simulink model "single_phase_half_wave_controlled_rectifier"  (R2024a)
settings: Solver=VariableStepAuto  StartTime=0.0  StopTime=0.1  RelTol=1e-3
libraries: spsRMSLib x3, spsCurrentMeasurementLib x2, spsVoltageMeasurementLib x2, spsMeanLib x1, spsSeriesRLCBranchLib x1, spsThyristorLib x1, spsACVoltageSourceLib x1, spspowerguiLib x1
settings Model: Creator=Asus  LastModifiedBy=Asus

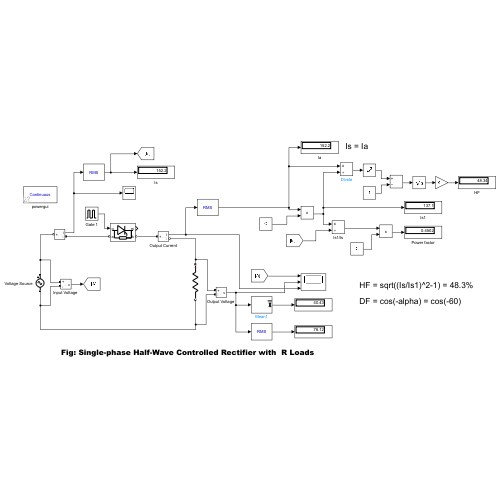
[thumbnail: Simulink's stored preview of the top-level diagram]
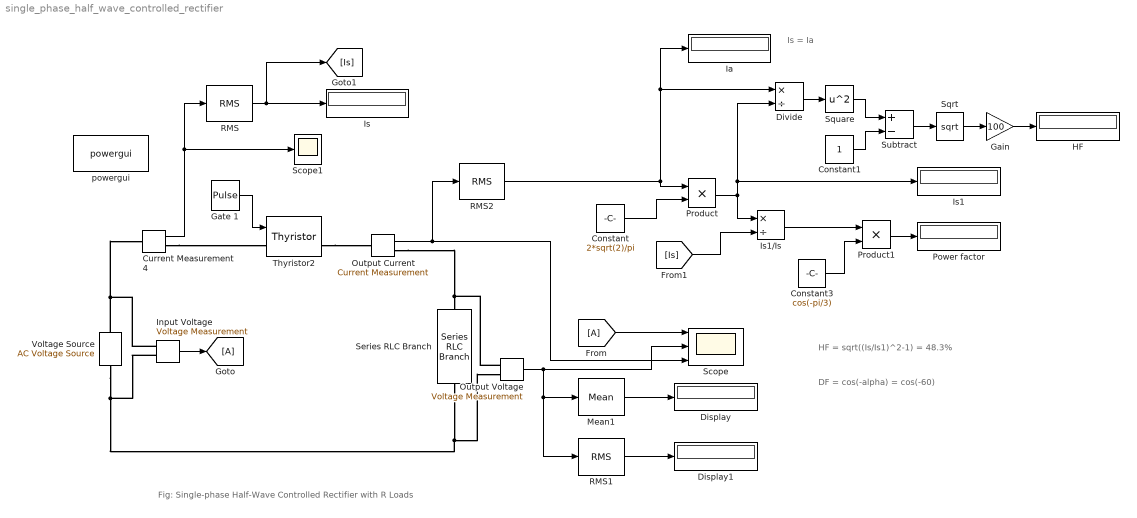
== system single_phase_half_wave_controlled_rectifier ==
  note: Is = Ia
  note: Fig: Single-phase Half-Wave Controlled Rectifier with R Loads
  note: HF = sqrt((Is/Is1)^2-1) = 48.3%
  note: DF = cos(-alpha) = cos(-60)
  Constant : Constant  Value=2*sqrt(2)/pi
  Constant1 : Constant
  Constant3 : Constant  Value=cos(-pi/3)
  Current Measurement4 : spsCurrentMeasurementLib/Current Measurement  PhasorSimulation=off  OutputType=Complex  PSBequivalent=0
  Display : Display
  Display1 : Display
  Divide : Product  Inputs=*/
  From : From
  Gain : Gain  Gain=100
  Gate 1 : DiscretePulseGenerator  PulseType=Time based  Period=1/60  PulseWidth=5  PhaseDelay=0.00277
  Goto : Goto
  HF : Display
  Ia : Display
  "Input Voltage " : spsVoltageMeasurementLib/Voltage Measurement  PhasorSimulation=off  OutputType=Complex  PSBequivalent=0
  Is : Display
  "Is1 " : Display
  Is1/Is : Product  Inputs=*/
  Mean1 : spsMeanLib/Mean  Freq=60  Vinit=0  Ts=0
  Output Current : spsCurrentMeasurementLib/Current Measurement  PhasorSimulation=off  OutputType=Complex  PSBequivalent=0
  "Output Voltage " : spsVoltageMeasurementLib/Voltage Measurement  PhasorSimulation=off  OutputType=Complex  PSBequivalent=0
  Power factor : Display
  Product : Product
  Product1 : Product
  RMS : spsRMSLib/RMS  TrueRMS=on  Freq=60  RMSInit=120  Ts=0
  RMS1 : spsRMSLib/RMS  TrueRMS=on  Freq=60  RMSInit=120  Ts=0
  RMS2 : spsRMSLib/RMS  TrueRMS=on  Freq=60  RMSInit=120  Ts=0
  Scope : Scope  NumInputPorts=3
  Scope1 : Scope
  Series RLC Branch : spsSeriesRLCBranchLib/Series RLC Branch  LConnTagsString=__new0  RConnTagsString=__new0  BranchType=R  Resistance=0.5  Inductance=6.5e-3  SetiL0=off  InitialCurrent=0  Capacitance=1e-6  Setx0=off  InitialVoltage=0  Measurements=None
  Sqrt : Sqrt
  Square : Math  Operator=square  SignedPower=on
  Subtract : Sum  Inputs=+-
  Thyristor2 : spsThyristorLib/Thyristor  Ron=0  Lon=0  Vf=0.1  IC=0  Rs=500  Cs=250e-9  Measurements=on
  Voltage Source : spsACVoltageSourceLib/AC Voltage Source  Amplitude=120*sqrt(2)  Phase=0  Frequency=60  SampleTime=0  Measurements=None  BusType=swing  Pref=10e3  Qref=0  Qmin=-inf  Qmax=+inf
  powergui : spspowerguiLib/powergui  Priority=1  SimulationMode=Continuous  SampleTime=50e-6  frequency=60  Iterations=50  frequencyindice=0  Pbase=100e6  ErrMax=1e-4  UnitsV=kV  UnitsW=MW  buscounter=0  FunctionMessages=off  echomessages=off  EnableUseOfTLC=off  CurrentSourceSwitches=off  DisableSnubberDevices=off  DisableRonSwitches=off  DisableVfSwitches=off  DisplayEquations=off  AutomaticDiscreteSolvers=off  SolverType=Tustin/Backward Euler (TBE)  Interpol=off  ExternalGateDelay=off  methode=off  Ts=100  x0status=blocks  SPID=on  SwTol=0  HookPort=off  NonlinearTolerance=0  nMaxIteration=15  ContinueOnMaxIteration=off  RestoreLinks=warning  ResistiveCurrentMeasurement=off  Frange=[0:2:500]  Ylog=off  Xlog=on  ShowGrid=off  save=off  variable=ZData  structure=p  ZoomFFT=off  StartTime=0.0  cycles=1  DisplayStyle=1  fundamental=60  FreqAxis=off  MaxFrequency=2500  frequencyindicesteady=1  RmsSteady=1  display=off
  wires:
  Divide/1 -> Square/1
  Mean1/1 -> Display/1
  Constant1/1 -> Subtract/2
  Gain/1 -> HF/1
  Product/1 -> Divide/2, "Is1 "/1, Is1/Is/1
  Constant3/1 -> Product1/2
  "Output Voltage "/1 -> Scope/2, RMS1/1, Mean1/1
  RMS/1 -> [Is], Is/1
  Gate 1/1 -> Thyristor2/1
  "Input Voltage "/1 -> Goto/1
  RMS2/1 -> Product/1, Ia/1, Divide/1
  [Is] -> Is1/Is/2
  Product1/1 -> Power factor/1
  Output Current/1 -> Scope/3, RMS2/1
  Current Measurement4/1 -> RMS/1, Scope1/1
  Is1/Is/1 -> Product1/1
  Constant/1 -> Product/2
  Sqrt/1 -> Gain/1
  Subtract/1 -> Sqrt/1
  Square/1 -> Subtract/1
  From/1 -> Scope/1
  RMS1/1 -> Display1/1
  connections:
  "Input Voltage "/LConn1 -- Voltage Source/RConn1 -- Current Measurement4/LConn1
  Voltage Source/LConn1 -- "Input Voltage "/LConn2 -- Series RLC Branch/RConn1 -- "Output Voltage "/LConn2
  Output Current/RConn1 -- "Output Voltage "/LConn1 -- Series RLC Branch/LConn1
  Thyristor2/RConn1 -- Output Current/LConn1
  Current Measurement4/RConn1 -- Thyristor2/LConn1
